simulink model "integrate_and_dump_team6"  (R2014a)
settings: Solver=ode45  StartTime=0.0  StopTime=100.0  RelTol=1e-3
libraries: commrandsrc2 x1, commnoisgen2 x1, commfilt2 x1
settings Model: Creator=alexw  LastModifiedBy=Renato
settings DataIOCC: SignalLoggingSaveFormat=ModelDataLogs
settings OptimizationCC: ExpressionDepthLimit=2147483647
settings DebuggingCC: UnderspecifiedInitializationDetection=Classic  FcnCallInpInsideContextMsg=UseLocalSettings  StateNameClashWarn=warning  StrictBusMsg=Warning
settings GRTTargetCC: CombineOutputUpdateFcns=off  GRTInterface=on

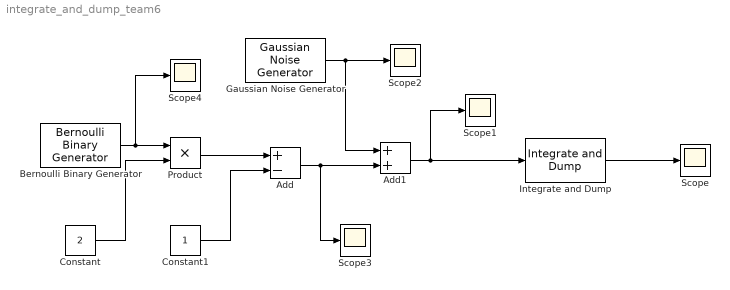
== system integrate_and_dump_team6 ==
  Add : Sum  Inputs=+-
  Add1 : Sum
  Bernoulli Binary Generator : commrandsrc2/Bernoulli Binary Generator  P=0.5  seed=61  Ts=1  frameBased=off  sampPerFrame=1  orient=off  outDataType=double
  Constant : Constant  Value=2
  Constant1 : Constant
  Gaussian Noise Generator : commnoisgen2/Gaussian Noise Generator  m=0  d=0.1  s=41  Ts=0.01  frameBased=off  sampPerFrame=1  orient=off  outDataType=double
  Integrate and Dump : commfilt2/Integrate and Dump  obssamples=100  offsetsamples=0  nodump=off  roundingMode=Floor  overflowMode=off
  Product : Product  RndMeth=Zero
  Scope{,1..4} (5 alike) : Scope
      Scope2 settings: SaveName=ScopeData2
      Scope3 settings: SaveName=ScopeData3
      Scope4 settings: SaveName=ScopeData4
  wires:
  Bernoulli Binary Generator/1 -> Product/1, Scope4/1
  Constant/1 -> Product/2
  Product/1 -> Add/1
  Constant1/1 -> Add/2
  Add/1 -> Add1/2, Scope3/1
  Gaussian Noise Generator/1 -> Add1/1, Scope2/1
  Add1/1 -> Integrate and Dump/1, Scope1/1
  Integrate and Dump/1 -> Scope/1
